simulink model "Fuel_level_harness"  (Simulink 7.7)
settings: Solver=FixedStepDiscrete  SolverMode=SingleTasking  StartTime=0.0  StopTime=100  FixedStep=0.1  RelTol=1e-3
InitFcn:
  | if signalbuilder('Fuel_level_harness/Signal_Builder','activegroup') == 1
  |   CD_FUEL_LEVEL_FUNCTION.DataType = 'uint8';
  |   CD_FUEL_LEVEL_FUNCTION.Value = 255;
  | else
  |   CD_FUEL_LEVEL_FUNCTION.DataType = 'uint8';
  |   CD_FUEL_LEVEL_FUNCTION.Value = 0;
  | end
  | 
  | if signalbuilder('Fuel_level_harness/Signal_Builder','activegroup') == 2
  |   CD_FUEL_WARN_FUNCTION.DataType = 'uint8';
  |   CD_FUEL_WARN_FUNCTION.Value = 255;
  | else
  |   CD_FUEL_WARN_FUNCTION.DataType = 'uint8';
  |   CD_FUEL_WARN_FUNCTION.Value = 0;
  | end
  | 
  | if signalbuilder('Fuel_level_harness/Signal_Builder','activegroup') == 6
  |   CD_FUEL_WARN_TIMEOUT.DataType = 'uint16';
  |   CD_FUEL_WARN_TIMEOUT.Value = 10;
  |   CD_FUEL_LEVEL_DEBOUNCE_OORL.DataType = 'uint16';
  |   CD_FUEL_LEVEL_DEBOUNCE_OORL.Value = 10;
  |   CD_FUEL_LEVEL_DEBOUNCE_OORH.DataType = 'uint16';
  |   CD_FUEL_LEVEL_DEBOUNCE_OORH.Value = 10;
  |   CD_FUEL_LEVEL_DEBOUNCE_NORMAL.DataType = 'uint16';
  |   CD_FUEL_LEVEL_DEBOUNCE_NORMAL.Value = 10;
  | else
  |   CD_FUEL_WARN_TIMEOUT.DataType = 'uint16';
  |   CD_FUEL_WARN_TIMEOUT.Value = 600;
  |   CD_FUEL_LEVEL_DEBOUNCE_OORL.DataType = 'uint16';
  |   CD_FUEL_LEVEL_DEBOUNCE_OORL.Value = 300;
  |   CD_FUEL_LEVEL_DEBOUNCE_OORH.DataType = 'uint16';
  |   CD_FUEL_LEVEL_DEBOUNCE_OORH.Value = 300;
  |   CD_FUEL_LEVEL_DEBOUNCE_NORMAL.DataType = 'uint16';
  |   CD_FUEL_LEVEL_DEBOUNCE_NORMAL.Value = 50;
  | end
undefined symbols (not defined in the file): CD_FUEL_LEVEL_FILTER_FAST_VALUE, CD_FUEL_LEVEL_FILTER_SLOW_VALUE, INACTIVE, MXGTW_FUELGAUGE, MXGTW_FUELSND, sigbuilder_block, srate100
libraries: MX_Library x4
settings Model: Creator=spencermindeman  LastModifiedBy=aliebel  CovMetricSettings=dctw  CovModelRefEnable=off
settings MATStruct: SampleTime=0.01  Offset=0  Priority=[1.0]
settings DataIOCC: LimitDataPoints=off  SaveOutput=off  SaveTime=off
settings OptimizationCC: BlockReduction=off  InlineParams=on  ExpressionFolding=off  StateBitsets=on  DataBitsets=on  UseTempVars=on  InitFltsAndDblsToZero=on  NoFixptDivByZeroProtection=on  EfficientFloat2IntCast=on  OptimizeModelRefInitCode=on
settings DebuggingCC: SaveWithParameterizedLinksMsg=none  MultiTaskDSMMsg=warning  MultiTaskCondExecSysMsg=none  IntegerOverflowMsg=none  ModelReferenceCSMismatchMessage=warning
settings HardwareCC: ProdBitPerInt=16  ProdBitPerPointer=16  ProdIntDivRoundTo=Floor  ProdEndianess=BigEndian  ProdWordSize=16  ProdHWDeviceType=Motorola HC12
settings ModelReferenceCC: ModelReferenceNumInstancesAllowed=Single
settings RTWCC: SystemTargetFile=ert.tlc  GenCodeOnly=on  TemplateMakefile=ert_default_tmf  Description=Real-Time Workshop Embedded Coder (no auto configuration)  GenerateReport=on  RetainRTWFile=on  ProcessScript=ert_make_rtw_hook  IncludeHyperlinkInReport=on  LaunchReport=on  IncludeERTFirstTime=on
settings RTWCC: CustomHeaderCode=|
  | #include "cpp_req_defines.h"
  | #include "hw_fin.h"
  | #include "cdata.h"
settings CodeAppCC: IgnoreCustomStorageClasses=off  DefineNamingRule=UpperCase
settings ERTTargetCC: TargetFcnLib=ansi_tfl_tmw.mat  FunctionExecutionProfile=off  MultiwordLength=2048  GenerateSampleERTMain=on  IncludeMdlTerminateFcn=off  SupportAbsoluteTime=off  SupportNonFinite=off  SupportComplex=off  PurelyIntegerCode=on  ERTCustomFileTemplate=gen_rtw_req_defines_h.tlc  GlobalDataDefinition=InSeparateSourceFile  GlobalDataReference=InSeparateHeaderFile  ConvertIfToSwitch=off

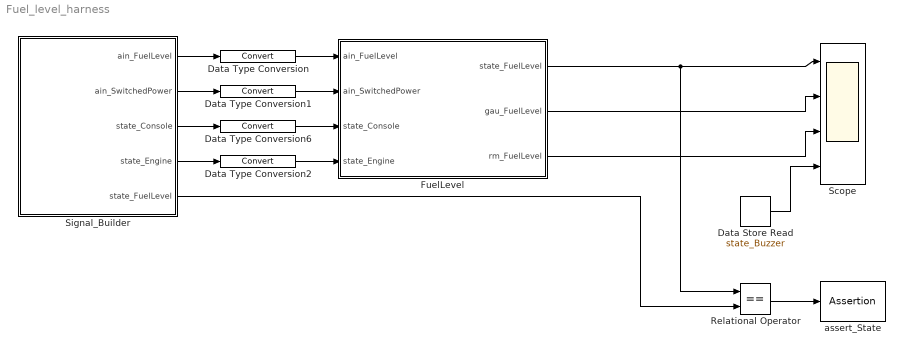
== system Fuel_level_harness ==
  Data Store Read : DataStoreRead  DataStoreName=state_Buzzer
  Data Type Conversion{,1..2,6} (4 alike) : DataTypeConversion
  FuelLevel : Subsystem  TreatAsAtomicUnit=on  SystemSampleTime=srate100  RTWFileName=mod_Inputs
      settings: RTWSystemCode=Function  RTWFileNameOpts=User specified
  Relational Operator : RelationalOperator  Operator===  OutDataTypeStr=boolean
  Scope : Scope  NumInputPorts=4
      settings: TimeRange=100  YMin=8~0~0~0  YMax=22~275~2000~17.5  MaxDataPoints=50000
  Signal_Builder : Subsystem  Tag=STV Subsys  LoadFcn=sigbuilder_block('load',[861 126 863.25 411 ]);  StartFcn=sigbuilder_block('start');  StopFcn=sigbuilder_block('stop');  ClipboardFcn=sigbuilder_block('clipboard');  mask(Sigbuilder block){}
      mask help: Sigbuilder GUI
      mask init:
      | if ~strcmp(get_param(bdroot(gcbh),'SimulationStatus'),'stopped') tuvar = sigbuilder_block('maskInit'); end
      settings: CopyFcn=sigbuilder_block('copy');  DeleteFcn=sigbuilder_block('delete');  ModelCloseFcn=sigbuilder_block('modelClose');  PreSaveFcn=sigbuilder_block('preSave');  NameChangeFcn=sigbuilder_block('namechange');  OpenFcn=sigbuilder_block('open',[-1200 -225 1200 849.75 ]);  CloseFcn=sigbuilder_block('close');
      mask Display: plot(0,0,100,100,[10,10,40,40,10],[80,20,20,80,80],[40,10],[50,50], [40,27,10],[65,72,56],[40,25,25,10],[28,28,43,43]);
  assert_State : Assertion  Enabled=off
  wires:
  Relational Operator/1 -> assert_State/1
  Data Type Conversion/1 -> FuelLevel/1(ain_FuelLevel)
  Data Type Conversion1/1 -> FuelLevel/2(ain_SwitchedPower)
  Data Type Conversion6/1 -> FuelLevel/3(state_Console)
  Signal_Builder/1(ain_FuelLevel) -> Data Type Conversion/1
  Signal_Builder/2(ain_SwitchedPower) -> Data Type Conversion1/1
  Signal_Builder/3(state_Console) -> Data Type Conversion6/1
  FuelLevel/1(state_FuelLevel) -> Scope/1, Relational Operator/1
  FuelLevel/2(gau_FuelLevel) -> Scope/2
  FuelLevel/3(rm_FuelLevel) -> Scope/3
  Signal_Builder/5(state_FuelLevel) -> Relational Operator/2
  Signal_Builder/4(state_Engine) -> Data Type Conversion2/1
  Data Type Conversion2/1 -> FuelLevel/4(state_Engine)
  Data Store Read/1 -> Scope/4

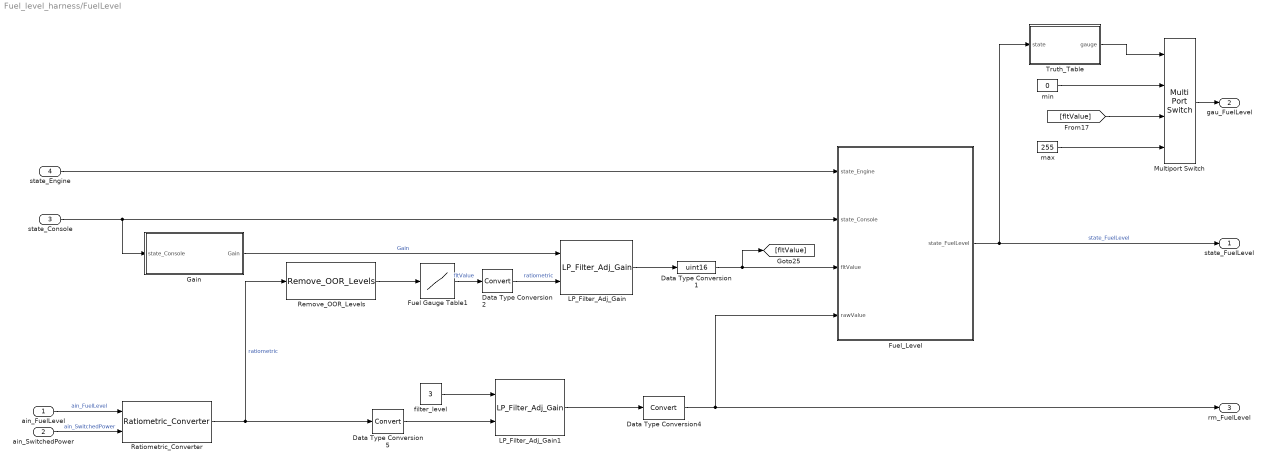
== system Fuel_level_harness/FuelLevel ==
  ain_FuelLevel : Inport  OutDataTypeStr=uint16
  ain_SwitchedPower : Inport  Port=2  OutDataTypeStr=uint16
  state_Console : Inport  Port=3
  state_Engine : Inport  Port=4
  Data Type Conversion1 : DataTypeConversion  OutDataTypeStr=uint16
  Data Type Conversion2 : DataTypeConversion
  Data Type Conversion4 : DataTypeConversion
  Data Type Conversion5 : DataTypeConversion
  Fuel Gauge Table1 : Lookup  InputValues=MXGTW_FUELSND  Table=MXGTW_FUELGAUGE  LookUpMeth=Use Input Nearest
      settings: AttributesFormatString=input = %<InputValues>\noutput = %<OutputValues>\nlookup = %<LookUpMeth>\nrounding = %<RndMeth>
  Fuel_Level : Stateflow chart  TreatAsAtomicUnit=on
  Gain : Stateflow chart  TreatAsAtomicUnit=on
  LP_Filter_Adj_Gain : MX_Library/LP_Filter_Adj_Gain  SystemSampleTime=-1
  LP_Filter_Adj_Gain1 : MX_Library/LP_Filter_Adj_Gain  SystemSampleTime=-1
  Multiport Switch : MultiPortSwitch  zeroidx=off  OutDataTypeStr=uint16
  Ratiometric_Converter : MX_Library/Ratiometric_Converter  SystemSampleTime=-1  multiplier=1000
  Remove_OOR_Levels : MX_Library/Remove_OOR_Levels  SystemSampleTime=-1  OORL_LEVEL=CD_FUEL_LEVEL_OORL  OORH_LEVEL=CD_FUEL_LEVEL_OORH
  Truth_Table : Stateflow chart  TreatAsAtomicUnit=on
  filter_level : Constant  Value=3  OutDataTypeStr=uint8
  max : Constant  Value=255  OutDataTypeStr=uint16
  min : Constant  Value=0  OutDataTypeStr=uint16  SampleTime=srate100
  state_FuelLevel : Outport
  gau_FuelLevel : Outport  Port=2
  rm_FuelLevel : Outport  Port=3
  wires:
  Fuel_Level/1(state_FuelLevel) -> state_FuelLevel/1, Truth_Table/1(state)  "state_FuelLevel"
  ain_SwitchedPower/1 -> Ratiometric_Converter/2  "ain_SwitchedPower"
  LP_Filter_Adj_Gain/1 -> Data Type Conversion1/1
  Gain/1(Gain) -> LP_Filter_Adj_Gain/1  "Gain"
  ain_FuelLevel/1 -> Ratiometric_Converter/1  "ain_FuelLevel"
  Ratiometric_Converter/1 -> Remove_OOR_Levels/1, Data Type Conversion5/1  "ratiometric"
  Data Type Conversion2/1 -> LP_Filter_Adj_Gain/2  "ratiometric"
  Multiport Switch/1 -> gau_FuelLevel/1
  min/1 -> Multiport Switch/2
  max/1 -> Multiport Switch/4
  LP_Filter_Adj_Gain1/1 -> Data Type Conversion4/1
  filter_level/1 -> LP_Filter_Adj_Gain1/1
  Data Type Conversion5/1 -> LP_Filter_Adj_Gain1/2
  state_Console/1 -> Gain/1(state_Console), Fuel_Level/2(state_Console)
  state_Engine/1 -> Fuel_Level/1(state_Engine)
  Truth_Table/1(gauge) -> Multiport Switch/1
  [fltValue] -> Multiport Switch/3
  Data Type Conversion4/1 -> rm_FuelLevel/1, Fuel_Level/4(rawValue)
  Fuel Gauge Table1/1 -> Data Type Conversion2/1  "fltValue"
  Data Type Conversion1/1 -> Fuel_Level/3(fltValue), [fltValue]
  Remove_OOR_Levels/1 -> Fuel Gauge Table1/1

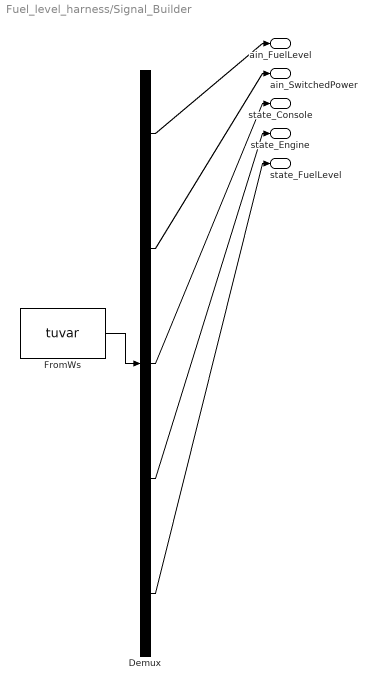
== system Fuel_level_harness/Signal_Builder ==
  Demux : Demux  Tag=STV Demux  Outputs=5
  FromWs : FromWorkspace  Tag=STV FromWs  VariableName=tuvar  SampleTime=0  SigBuilderData=DataTag0  VnvData=DataTag1
      SigBuilderData=|
      | common.afterFinalStr = 'Extrapolate'
      | common.sampleTime = 0
      | dataSet(1).timeRange = [0 100]
      | dataSet(1).name = 'T1-NON_FUNC'
      | dataSet(2).timeRange = [0 100]
      | dataSet(2).name = 'T2-OOR'
      | dataSet(3).timeRange = [0 100]
      | dataSet(3).name = 'T3-LOW'
      | dataSet(4).timeRange = [0 100]
      | dataSet(4).name = 'T4-GAIN'
      | dataSet(5).timeRange = [0 100]
      | dataSet(5).name = 'T5-GAIN2'
      | dataSet(6).timeRange = [0 100]
      | dataSet(6).name = 'T6-Fill_Warning'
      | dataSet(7).timeRange = [0 100]
      | dataSet(7).name = 'T7-Fill_Warning1'
      | sbobj.Groups(1).Name = 'T1-NON_FUNC'
      | sbobj.Groups(1).Signals(1).Name = 'ain_FuelLevel'
      | sbobj.Groups(1).Signals(1).XData = [0 100]
      | sbobj.Groups(1).Signals(1).YData = [0 0]
      | sbobj.Groups(1).Signals(2).Name = 'ain_SwitchedPower'
      | sbobj.Groups(1).Signals(2).XData = [0 100]
      | sbobj.Groups(1).Signals(2).YData = [0 0]
      | sbobj.Groups(1).Signals(3).Name = 'state_Console'
      | sbobj.Groups(1).Signals(3).XData = [0 100]
      | sbobj.Groups(1).Signals(3).YData = [0 0]
      | sbobj.Groups(1).Signals(4).Name = 'state_Engine'
      | sbobj.Groups(1).Signals(4).XData = [0 100]
      | sbobj.Groups(1).Signals(4).YData = [0 0]
      | sbobj.Groups(1).Signals(5).Name = 'state_FuelLevel'
      | sbobj.Groups(1).Signals(5).XData = [0 100]
      | sbobj.Groups(1).Signals(5).YData = [8 8]
      | sbobj.Groups(2).Name = 'T2-OOR'
      | sbobj.Groups(2).Signals(1).Name = 'ain_FuelLevel'
      | sbobj.Groups(2).Signals(1).XData = [0 1.2 1.2 6 6 8.4 8.4 43.9 43.9 44.6 44.6 47.3 47.3 53.2 53.2 55.8 55.8 57.2 57.2 89.4 89.4 90.2 90.2 91.4 91.4 100]
      | sbobj.Groups(2).Signals(1).YData = [100 100 0 0 100 100 0 0 100 100 0 0 100 100 1000 1000 100 100 1000 1000 10 10 1000 1000 100 100]
      | sbobj.Groups(2).Signals(2).Name = 'ain_SwitchedPower'
      | sbobj.Groups(2).Signals(2).XData = [0 100]
      | sbobj.Groups(2).Signals(2).YData = [500 500]
      | sbobj.Groups(2).Signals(3).Name = 'state_Console'
      | sbobj.Groups(2).Signals(3).XData = [0 100]
      | sbobj.Groups(2).Signals(3).YData = [0 0]
      | sbobj.Groups(2).Signals(4).Name = 'state_Engine'
      | sbobj.Groups(2).Signals(4).XData = [0 100]
      | sbobj.Groups(2).Signals(4).YData = [0 0]
      | sbobj.Groups(2).Signals(5).Name = 'state_FuelLevel'
      | sbobj.Groups(2).Signals(5).XData = [0 40.1 40.1 52.4 52.4 88.1 88.1 96.6 96.6 100]
      | sbobj.Groups(2).Signals(5).YData = [8 8 22 22 8 8 21 21 8 8]
      | sbobj.Groups(3).Name = 'T3-LOW'
      | sbobj.Groups(3).Signals(1).Name = 'ain_FuelLevel'
      | sbobj.Groups(3).Signals(1).XData = [0 0.9 0.9 4.2 4.2 45.5 45.5 47.3 47.3 50 50 59.9 60.9 60.9 96.6 96.6 100]
      | sbobj.Groups(3).Signals(1).YData = [500 500 300 300 500 500 195 195 500 500 340 292.48 297.655062344 500 500 1000 1000]
      | sbobj.Groups(3).Signals(2).Name = 'ain_SwitchedPower'
      | sbobj.Groups(3).Signals(2).XData = [0 100]
      | sbobj.Groups(3).Signals(2).YData = [500 500]
      | sbobj.Groups(3).Signals(3).Name = 'state_Console'
      | sbobj.Groups(3).Signals(3).XData = [0 100]
      | sbobj.Groups(3).Signals(3).YData = [0 0]
      | sbobj.Groups(3).Signals(4).Name = 'state_Engine'
      | sbobj.Groups(3).Signals(4).XData = [0 100]
      | sbobj.Groups(3).Signals(4).YData = [0 0]
      | sbobj.Groups(3).Signals(5).Name = 'state_FuelLevel'
      | sbobj.Groups(3).Signals(5).XData = [0 30.3 30.3 59.9 59.9 92.3 92.3 100]
      | sbobj.Groups(3).Signals(5).YData = [8 8 9 9 8 8 9 9]
      | sbobj.Groups(4).Name = 'T4-GAIN'
      | sbobj.Groups(4).Signals(1).Name = 'ain_FuelLevel'
      | sbobj.Groups(4).Signals(1).XData = [0 100]
      | sbobj.Groups(4).Signals(1).YData = [0 1000]
      | sbobj.Groups(4).Signals(2).Name = 'ain_SwitchedPower'
      | sbobj.Groups(4).Signals(2).XData = [0 100]
      | sbobj.Groups(4).Signals(2).YData = [500 500]
      | sbobj.Groups(4).Signals(3).Name = 'state_Console'
      | sbobj.Groups(4).Signals(3).XData = [0 100]
      | sbobj.Groups(4).Signals(3).YData = [0 0]
      | sbobj.Groups(4).Signals(4).Name = 'state_Engine'
      | sbobj.Groups(4).Signals(4).XData = [0 100]
      | sbobj.Groups(4).Signals(4).YData = [0 0]
      | sbobj.Groups(4).Signals(5).Name = 'state_FuelLevel'
      | sbobj.Groups(4).Signals(5).XData = [0 68.7 68.7 100]
      | sbobj.Groups(4).Signals(5).YData = [8 8 9 9]
      | sbobj.Groups(5).Name = 'T5-GAIN2'
      | sbobj.Groups(5).Signals(1).Name = 'ain_FuelLevel'
      | sbobj.Groups(5).Signals(1).XData = [0 100]
      | sbobj.Groups(5).Signals(1).YData = [0 1000]
      | sbobj.Groups(5).Signals(2).Name = 'ain_SwitchedPower'
      | sbobj.Groups(5).Signals(2).XData = [0 100]
      | sbobj.Groups(5).Signals(2).YData = [500 500]
      | sbobj.Groups(5).Signals(3).Name = 'state_Console'
      | sbobj.Groups(5).Signals(3).XData = [0 100]
      | sbobj.Groups(5).Signals(3).YData = [1 1]
      | sbobj.Groups(5).Signals(4).Name = 'state_Engine'
      | sbobj.Groups(5).Signals(4).XData = [0 100]
      | sbobj.Groups(5).Signals(4).YData = [0 0]
      | sbobj.Groups(5).Signals(5).Name = 'state_FuelLevel'
      | sbobj.Groups(5).Signals(5).XData = [0 91.7 100]
      | sbobj.Groups(5).Signals(5).YData = [8 8 8]
      | sbobj.Groups(6).Name = 'T6-Fill_Warning'
      | sbobj.Groups(6).Signals(1).Name = 'ain_FuelLevel'
      | sbobj.Groups(6).Signals(1).XData = [0 2 2 5.4 5.4 6.8 7.8 10 10 18.4 28.2 40 40 90 100]
      | sbobj.Groups(6).Signals(1).YData = [50 50 0 0 540 520 1000 1000 500 500 200 180 500 50 50]
      | sbobj.Groups(6).Signals(2).Name = 'ain_SwitchedPower'
      | sbobj.Groups(6).Signals(2).XData = [0 100]
      | sbobj.Groups(6).Signals(2).YData = [500 500]
      | sbobj.Groups(6).Signals(3).Name = 'state_Console'
      | sbobj.Groups(6).Signals(3).XData = [0 13.4 13.4 14.2 14.2 100]
      | sbobj.Groups(6).Signals(3).YData = [0 0 1 1 0 0]
      | sbobj.Groups(6).Signals(4).Name = 'state_Engine'
      | sbobj.Groups(6).Signals(4).XData = [0 15.6 15.6 16.4 16.4 100]
      | sbobj.Groups(6).Signals(4).YData = [1 1 2 2 1 1]
      | sbobj.Groups(6).Signals(5).Name = 'state_FuelLevel'
      | sbobj.Groups(6).Signals(5).XData = [0 91.7 100]
      | sbobj.Groups(6).Signals(5).YData = [8 8 8]
      | sbobj.Groups(7).Name = 'T7-Fill_Warning1'
      | sbobj.Groups(7).Signals(1).Name = 'ain_FuelLevel'
      | sbobj.Groups(7).Signals(1).XData = [0 10 10 18.4 28.2 40 40 90 100]
      | sbobj.Groups(7).Signals(1).YData = [240 240 500 500 170 180 500 50 50]
      | sbobj.Groups(7).Signals(2).Name = 'ain_SwitchedPower'
      | sbobj.Groups(7).Signals(2).XData = [0 100]
      | sbobj.Groups(7).Signals(2).YData = [500 500]
      | sbobj.Groups(7).Signals(3).Name = 'state_Console'
      | sbobj.Groups(7).Signals(3).XData = [0 32.4 32.4 33 33 100]
      | sbobj.Groups(7).Signals(3).YData = [0 0 1 1 0 0]
      | sbobj.Groups(7).Signals(4).Name = 'state_Engine'
      | sbobj.Groups(7).Signals(4).XData = [0 96.8 96.8 97.6 97.6 100]
      | sbobj.Groups(7).Signals(4).YData = [1 1 2 2 1 1]
      | sbobj.Groups(7).Signals(5).Name = 'state_FuelLevel'
      | sbobj.Groups(7).Signals(5).XData = [0 91.7 100]
      | sbobj.Groups(7).Signals(5).YData = [8 8 8]
  ain_FuelLevel : Outport  Tag=STV Outport
  ain_SwitchedPower : Outport  Tag=STV Outport  Port=2
  state_Console : Outport  Tag=STV Outport  Port=3
  state_Engine : Outport  Tag=STV Outport  Port=4
  state_FuelLevel : Outport  Tag=STV Outport  Port=5
  wires:
  FromWs/1 -> Demux/1
  Demux/1 -> ain_FuelLevel/1
  Demux/2 -> ain_SwitchedPower/1
  Demux/3 -> state_Console/1
  Demux/4 -> state_Engine/1
  Demux/5 -> state_FuelLevel/1

== stateflow chart FuelLevel/Fuel_Level ==
  state FuelFillWarning [parallel]
    settings: executionOrder=2
    state Inactive
    state Active
      state Intermittant_Beep
        en:
        beep_Delay = (255c - fltValue)/8c;
      state Armed
        en:
        start_FuelLevel = fltValue;
        previous_Delay = 31;
        delay_Limit = 0;
      state Continuous
        en:
        state_Buzzer = CONTINUOUS_BEEP;
        ex:
        state_Buzzer = NO_BEEP;
      (default) -> Armed
      Intermittant_Beep -> (junction 24) [order 2] : [after(uint8(beep_Delay),tick)]
      Armed -> Intermittant_Beep : [fltValue >...
          | (start_FuelLevel + CD_FUEL_WARN_DELTA)]
      (junction 24) -> (junction 25) : {
          | state_Buzzer = SINGLE_SHORT_BEEP;
          | }
      (junction 25) -> (junction 26) [order 1] : [uint8(beep_Delay) == previous_Delay]
      (junction 25) -> (junction 27) [order 2] : {
          | previous_Delay = uint8(beep_Delay);
          | delay_Limit = 0;
          | }
      (junction 26) -> (junction 28) : {
          | delay_Limit+= uint8(beep_Delay);
          | }
      Intermittant_Beep -> Armed [order 3] : [delay_Limit > CD_FUEL_WARN_TIMEOUT]
      (junction 27) -> Intermittant_Beep
      (junction 28) -> (junction 27)
      Intermittant_Beep -> Continuous [order 1] : [beep_Delay == 0]
      Continuous -> Armed : [after(CD_FUEL_WARN_TIMEOUT,tick)]
    (default) -> Inactive
    Active -> Inactive : [state_Console != INACTIVE...
        | || state_Engine != ENGINE_NOT_RUNNING...
        | || state_FuelLevel == OORL...
        | || state_FuelLevel == OORH]
    Inactive -> Active : [CD_FUEL_WARN_FUNCTION != NON_FUNCTIONAL...
        | && state_Console == INACTIVE...
        | && state_Engine == ENGINE_NOT_RUNNING...
        | && state_FuelLevel != OORL...
        | && state_FuelLevel != OORH]
  state Monitor [parallel]
    settings: executionOrder=1
    state NON_FUNCTIONAL
      en:state_FuelLevel = NORMAL;
    state NORMAL
      state NORMAL
        state DEBOUNCE
          en:debounceCount = 0;
          du:debounceCount++;
        state NORMAL
          en:state_FuelLevel = NORMAL;
        (default) -> Monitor.NORMAL.NORMAL.DEBOUNCE
        Monitor.NORMAL.NORMAL.DEBOUNCE -> Monitor.NORMAL.NORMAL.NORMAL : [(debounceCount >= CD_FUEL_LEVEL_DEBOUNCE_NORMAL)...
            | || (state_FuelLevel == NORMAL)]
      state LOW
        state LOW
          en:state_FuelLevel = LOW;
        state DEBOUNCE
          en:debounceCount = 0;
          du:debounceCount++;
        Monitor.NORMAL.LOW.DEBOUNCE -> Monitor.NORMAL.LOW.LOW : [(debounceCount >= CD_FUEL_LEVEL_DEBOUNCE_LOW)...
            | || (state_FuelLevel == LOW)]
        (default) -> Monitor.NORMAL.LOW.DEBOUNCE
      (default) -> Monitor.NORMAL.NORMAL
      Monitor.NORMAL.LOW -> Monitor.NORMAL.NORMAL : [(fltValue > CD_FUEL_RESET_VALUE)]
      Monitor.NORMAL.NORMAL -> Monitor.NORMAL.LOW : [(fltValue <= CD_FUEL_LEVEL_LOW)]
    state OORL
      state NORMAL
        en:state_FuelLevel = OORL;
      state DEBOUNCE
        en:debounceCount = 0;
        du:debounceCount++;
      Monitor.OORL.DEBOUNCE -> Monitor.OORL.NORMAL : [(debounceCount >= CD_FUEL_LEVEL_DEBOUNCE_OORL)...
          | || (state_FuelLevel == OORL)]
      (default) -> Monitor.OORL.DEBOUNCE
    state OORH
      state DEBOUNCE
        en:debounceCount = 0;
        du:debounceCount++;
      state NORMAL
        en:state_FuelLevel = OORH;
      (default) -> Monitor.OORH.DEBOUNCE
      Monitor.OORH.DEBOUNCE -> Monitor.OORH.NORMAL : [(debounceCount >= CD_FUEL_LEVEL_DEBOUNCE_OORH)...
          | || (state_FuelLevel == OORH)]
    (default) -> NON_FUNCTIONAL
    NON_FUNCTIONAL -> Monitor.NORMAL : [(CD_FUEL_LEVEL_FUNCTION != NON_FUNCTIONAL)]
    Monitor.NORMAL -> OORL [order 2] : [(rawValue <= CD_FUEL_LEVEL_OORL)]
    OORL -> Monitor.NORMAL : [(rawValue > CD_FUEL_LEVEL_OORL)]
    Monitor.NORMAL -> OORH [order 1] : [(rawValue >= CD_FUEL_LEVEL_OORH)]
    OORH -> Monitor.NORMAL : [(rawValue < CD_FUEL_LEVEL_OORH)]
  data: state_Engine input uint8; state_Console input uint8; fltValue input uint16; rawValue input uint16; state_FuelLevel output uint8; CD_FUEL_LEVEL_FUNCTION parameter uint8; CD_FUEL_LEVEL_LOW parameter uint16; CD_FUEL_LEVEL_OORL parameter uint16; CD_FUEL_LEVEL_OORH parameter uint16; CD_FUEL_LEVEL_DEBOUNCE_NORMAL parameter uint16; CD_FUEL_LEVEL_DEBOUNCE_OORL parameter uint16; CD_FUEL_LEVEL_DEBOUNCE_OORH parameter uint16; CD_FUEL_LEVEL_DEBOUNCE_LOW parameter uint16; CD_FUEL_RESET_VALUE parameter uint8; debounceCount local uint16 =0; OORH parameter uint8 =21; OORL parameter uint8 =22; NON_FUNCTIONAL parameter uint8 =255; NORMAL parameter uint8 =8; LOW parameter uint8 =9; CD_FUEL_WARN_DELTA parameter uint16; CD_FUEL_WARN_FUNCTION parameter uint8; CD_FUEL_WARN_TIMEOUT parameter uint16; ENGINE_NOT_RUNNING parameter uint8; INACTIVE parameter uint8; NO_BEEP parameter uint8; beep_Delay local uint16; delay_Limit local uint16; previous_Delay local uint16; start_FuelLevel local uint16; state_Buzzer data_store_memory double; CONTINUOUS_BEEP parameter uint8; SINGLE_SHORT_BEEP parameter uint8

== stateflow chart FuelLevel/Gain ==
  (junction 96) -> (junction 97) [order 1] : [(state_Console != INACTIVE)]
  (junction 97) -> (junction 99) : {
      | Gain = CD_FUEL_LEVEL_FILTER_SLOW_VALUE;
      | }
  (junction 99) -> (junction 98)
  (junction 96) -> (junction 98) [order 2] : {
      | Gain = CD_FUEL_LEVEL_FILTER_FAST_VALUE;
      | }
  (default) -> (junction 96)
  data: state_Console input uint8; Gain output uint8; CD_FUEL_LEVEL_FILTER_SLOW_VALUE parameter uint8; CD_FUEL_LEVEL_FILTER_FAST_VALUE parameter uint8; INACTIVE parameter uint8

== matlab function FuelLevel/Truth_Table ==
  data: state input uint8; gauge output uint8
function gauge = fcn(state)

aVarTruthTableCondition_1 = false;
aVarTruthTableCondition_2 = false;


% OORH

aVarTruthTableCondition_1 = logical(state == 21);

% OORL

aVarTruthTableCondition_2 = logical(state == 22);

if (aVarTruthTableCondition_1)
    aFcnTruthTableAction_3();
elseif (aVarTruthTableCondition_2)
    aFcnTruthTableAction_1();
else % Default
    aFcnTruthTableAction_2();
end

function aFcnTruthTableAction_1()

% Gauge min

gauge = uint8(1);

function aFcnTruthTableAction_2()

% Gauge current

gauge = uint8(2);

function aFcnTruthTableAction_3()

% Gauge max

gauge = uint8(3);
